simulink model "FMUimportTestDymolaFMU"  (R2025a)
settings: Solver=ode15s  StartTime=0.0  StopTime=30  RelTol=1e-6
settings Model: Creator=vanfr  LastModifiedBy=vanfr

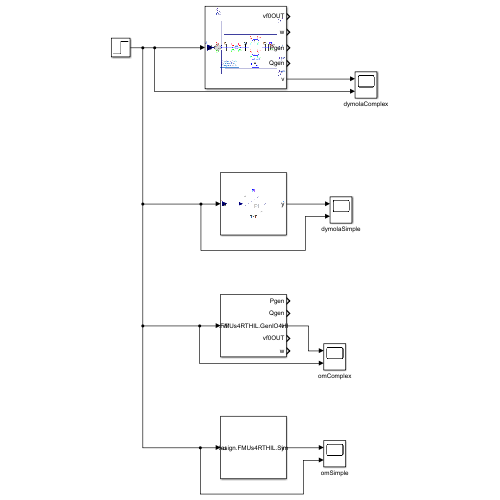
[thumbnail: Simulink's stored preview of the top-level diagram]
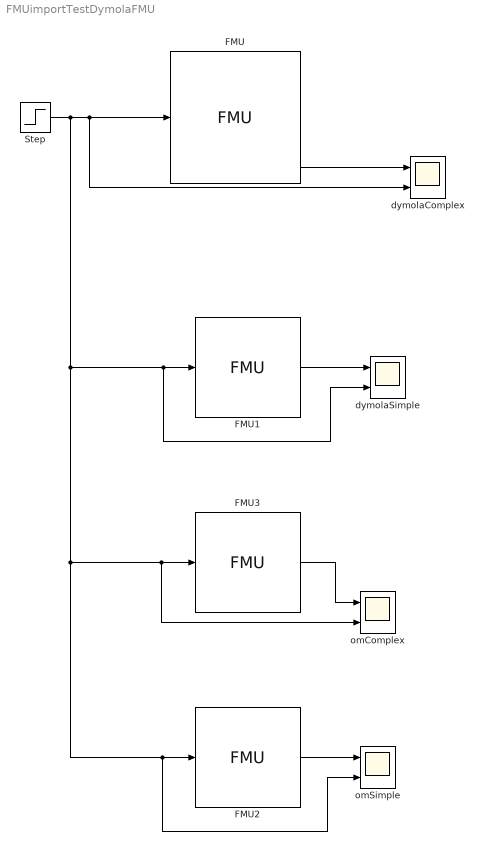
== system FMUimportTestDymolaFMU ==
  FMU : FMU  FMUName=PSSDesign_FMUs4RTHIL_GenIO4HILinNetwork.fmu  FMUMode=ModelExchange  FMUInitializeEnumObject=off  SysData=struct('S_b',100000000.0,'fn',60)  B1=struct('V_b',400000.0,'P_0',1000000.0,'Q_0',0,'v_0',1,'angle_0',0,'displayPF',boolean(false))  B2=struct('V_b',400000.0,'P_0',1000000.0,'Q_0',0,'v_0',1,'angle_0',0,'displayPF',boolean(false))  B3=struct('V_b',400000.0,'P_0',1000000.0,'Q_0',0,'v_0',1,'angle_0',0,'displayPF',boolean(false))  G1=struct('V_b',400000.0,'P_0',1997999999.9936,'Q_0',967924969.90658,'v_0',1,'angle_0',0.49467717698916,'displayPF',boolean(false),'machine',struct('displayPF',boolean(false),'Sn',2220000000.0,'Vn',400000,'ra',0.003,'x1d',0.3,'M',7,'xd',1.81,'xq',1.76,'x1q',0.65,'x2d',0.23,'x2q',0.25,'T1d0',8,'T1q0',1,'T2d0',0.03,'T2q0',0.07,'Taa',0.002),'gainVf0',struct('k',-1))  transformer=struct('V_b',400000,'Sn',2220000000.0,'Vn',400000,'rT',0,'xT',0.15,'m_2',1.0,'displayPF',boolean(false))  pwLine1=struct('R',0,'X',0.02252252252252252,'G',0,'B',0,'S_b',100000000.0,'displayPF',boolean(false))  pwLine2=struct('R',0,'X',0.041891891891891894,'G',0,'B',0,'S_b',100000000.0,'displayPF',boolean(false))  infiniteBus=struct('V_b',400000.0,'P_0',-1998000000,'Q_0',87066000,'v_0',0.90081,'angle_0',0,'displayPF',boolean(false))  mask(PSSDesign.FMUs4RTHIL.GenIO4HILinNetwork [Model Exchange, v2.0]){}
      settings: MultithreadedSim=off
      mask Display:
      | if (exist([Simulink.fileGenControl('get','CacheFolder') '\slprj\_fmu\8d1074ac16570a03b4f9af9a0dd0adcb\PSSDesign_FMUs4RTHIL_GenIO4HILinNetwork\model.png'],'file'))
      |     image([Simulink.fileGenControl('get','CacheFolder') '\slprj\_fmu\8d1074ac16570a03b4f9af9a0dd0adcb\PSSDesign_FMUs4RTHIL_GenIO4HILinNetwork\model.png']);
      | else
      |     disp('PSSDesign.FMUs4RTHIL.GenIO4HILinNetwork');
      | end
      | port_label('output',1,'vf0OUT');
      | port_label('output',2,'w');
      | port_label('output',3,'Pgen');
      | port_label('output',4,'Qgen');
      | port_label('output',5,'v');
      | port_label('input',1,'vf');
  FMU1 : FMU  FMUName=PSSDesign_FMUs4RTHIL_SimplePI.fmu  FMUMode=ModelExchange  FMUInitializeEnumObject=off  PI=struct('k',1,'T',0.1,'x_start',0,'y_start',0)  mask(PSSDesign.FMUs4RTHIL.SimplePI [Model Exchange, v2.0]){}
      settings: MultithreadedSim=off
      mask Display:
      | if (exist([Simulink.fileGenControl('get','CacheFolder') '\slprj\_fmu\9ffa2c13b0a163024a908bd4c4f9bfa6\PSSDesign_FMUs4RTHIL_SimplePI\model.png'],'file'))
      |     image([Simulink.fileGenControl('get','CacheFolder') '\slprj\_fmu\9ffa2c13b0a163024a908bd4c4f9bfa6\PSSDesign_FMUs4RTHIL_SimplePI\model.png']);
      | else
      |     disp('PSSDesign.FMUs4RTHIL.SimplePI');
      | end
      | port_label('output',1,'y');
      | port_label('input',1,'u');
  FMU2 : FMU  FMUName=SimplePI.fmu  FMUMode=ModelExchange  FMUInitializeEnumObject=off  PI=struct('T',0.1,'k',1.0,'x_start',0.0,'y_start',0.0,'initType',int32(1))  mask(PSSDesign.FMUs4RTHIL.SimplePI [Model Exchange, v2.0]){}
      settings: MultithreadedSim=off
      mask Display:
      | disp('PSSDesign.FMUs4RTHIL.SimplePI');
      | port_label('output',1,'y');
      | port_label('input',1,'u');
  FMU3 : FMU  FMUName=GenIO4HILinNetwork.fmu  FMUMode=ModelExchange  FMUInitializeEnumObject=off  B1=struct('P_0',1e6,'Q_0',0.0,'S_b',0,'V_b',4e5,'angle_0',0.0,'fn',0,'v_0',1.0,'displayPF',boolean(false),'enableP_0',boolean(0),'enableQ_0',boolean(0),'enableS_b',boolean(0),'enableV_b',boolean(0),'enableangle_0',boolean(0),'enabledisplayPF',boolean(0),'enablefn',boolean(0),'enablev_0',boolean(0))  B2=struct('P_0',1e6,'Q_0',0.0,'S_b',0,'V_b',4e5,'angle_0',0.0,'fn',0,'v_0',1.0,'displayPF',boolean(false),'enableP_0',boolean(0),'enableQ_0',boolean(0),'enableS_b',boolean(0),'enableV_b',boolean(0),'enableangle_0',boolean(0),'enabledisplayPF',boolean(0),'enablefn',boolean(0),'enablev_0',boolean(0))  B3=struct('P_0',1e6,'Q_0',0.0,'S_b',0,'V_b',4e5,'angle_0',0.0,'fn',0,'v_0',1.0,'displayPF',boolean(false),'enableP_0',boolean(0),'enableQ_0',boolean(0),'enableS_b',boolean(0),'enableV_b',boolean(0),'enableangle_0',boolean(0),'enabledisplayPF',boolean(0),'enablefn',boolean(0),'enablev_0',boolean(0))  G1=struct('P_0',1.9979999999936e9,'Q_0',9.6792496990658e8,'S_b',0,'V_b',4e5,'angle_0',0.49467717698916,'fn',0,'gainVf0',struct('k',-1.0,'u',0),'machine',struct('D',0,'M',7.0,'P_0',0,'Q_0',0,'S_b',0,'Sn',2.22e9,'T1d0',8.0,'T1q0',1.0,'T2d0',0.03,'T2q0',0.07,'Taa',0.002,'V_b',0,'Vn',4e5,'angle_0',0,'fn',0,'pm',0,'pm0',0,'ra',0.003,'v_0',0,'vf0',0,'x1d',0.3,'x1q',0.65,'x2d',0.23,'x2q',0.25,'xd',1.81,'xq',1.76,'displayPF',boolean(false),'enableP_0',boolean(0),'enableQ_0',boolean(0),'enableS_b',boolean(0),'enableV_b',boolean(0),'enableangle_0',boolean(0),'enabledisplayPF',boolean(0),'enablefn',boolean(0),'enablev_0',boolean(0)),'v_0',1.0,'vf0OUT',0,'displayPF',boolean(false),'enableP_0',boolean(0),'enableQ_0',boolean(0),'enableS_b',boolean(0),'enableV_b',boolean(0),'enableangle_0',boolean(0),'enabledisplayPF',boolean(0),'enablefn',boolean(0),'enablev_0',boolean(0))  SysData=struct('S_b',1e8,'fn',60.0)  infiniteBus=struct('P_0',-1.998e9,'Q_0',8.7066e7,'S_b',0,'V_b',4e5,'angle_0',0.0,'fn',0,'v_0',0.90081,'displayPF',boolean(false),'enableP_0',boolean(0),'enableQ_0',boolean(0),'enableS_b',boolean(0),'enableV_b',boolean(0),'enableangle_0',boolean(0),'enabledisplayPF',boolean(0),'enablefn',boolean(0),'enablev_0',boolean(0))  pwFault=struct('R',0.0,'X',4.5045045045045046e-4,'t1',30.5,'t2',30.57)  pwLine1=struct('B',0.0,'G',0.0,'R',0.0,'S_b',1e8,'X',0.02252252252252252,'t1',1e60,'t2',1e60,'opening',int32(0),'displayPF',boolean(false))  pwLine2=struct('B',0.0,'G',0.0,'R',0.0,'S_b',1e8,'X',0.041891891891891894,'t1',1e60,'t2',1e60,'opening',int32(0),'displayPF',boolean(false))  transformer=struct('S_b',0,'Sn',2.22e9,'V_b',4e5,'Vn',4e5,'m_2',1.0,'rT',0.0,'xT',0.15,'displayPF',boolean(false))  mask(PSSDesign.FMUs4RTHIL.GenIO4HILinNetwork [Model Exchange, v2.0]){}
      settings: MultithreadedSim=off
      mask Display:
      | disp('PSSDesign.FMUs4RTHIL.GenIO4HILinNetwork');
      | port_label('output',1,'Pgen');
      | port_label('output',2,'Qgen');
      | port_label('output',3,'v');
      | port_label('output',4,'vf0OUT');
      | port_label('output',5,'w');
      | port_label('input',1,'vf');
  Step : Step  Time=5  After=0.005  SampleTime=0
  dymolaComplex : Scope  NumInputPorts=2
      settings: ActiveDisplayYMinimum=0.99967188000922191  ActiveDisplayYMaximum=1.0029530798750124
  dymolaSimple : Scope  NumInputPorts=2
      settings: ActiveDisplayYMinimum=-0.15687499999999979  ActiveDisplayYMaximum=1.4118749999999984
  omComplex : Scope  NumInputPorts=2
      settings: ActiveDisplayYMinimum=0.99939370866717991  ActiveDisplayYMaximum=1.0029211966765528  DataLoggingVariableName=ScopeData2
  omSimple : Scope  NumInputPorts=2
      settings: ActiveDisplayYMinimum=-0.15687499999999974  ActiveDisplayYMaximum=1.411874999999998  DataLoggingVariableName=ScopeData3
  wires:
  FMU/5 -> dymolaComplex/1
  FMU1/1 -> dymolaSimple/1
  FMU2/1 -> omSimple/1
  Step/1 -> omSimple/2, FMU2/1, omComplex/2, FMU3/1, dymolaSimple/2, FMU1/1, dymolaComplex/2, FMU/1
  FMU3/3 -> omComplex/1
